simulink model "sla_tf2filter"  (R2015b)
settings: Solver=FixedStepDiscrete  SolverMode=SingleTasking  StartTime=0.0  StopTime=10.0  RelTol=1e-3
undefined symbols (not defined in the file or in its folder): dfilt
libraries: simulink x1, dsparch4 x1
settings Model: Creator=at-mt  LastModifiedBy=amatsumo
settings DataIOCC: SaveFormat=Array  SignalLoggingSaveFormat=ModelDataLogs  SaveOutput=off  SignalLogging=off  SaveTime=off
settings OptimizationCC: BlockReduction=off  ConditionallyExecuteInputs=off  DefaultParameterBehavior=Inlined  ExpressionDepthLimit=2147483647
settings DebuggingCC: AlgebraicLoopMsg=error  UnderspecifiedInitializationDetection=Classic  MergeDetectMultiDrivingBlocksExec=none  SolverPrmCheckMsg=warning  SingleTaskRateTransMsg=error  FcnCallInpInsideContextMsg=UseLocalSettings  StateNameClashWarn=warning
settings HardwareCC: ProdBitPerPointer=32  ProdLargestAtomicFloat=None  ProdIntDivRoundTo=Undefined  ProdEndianess=Unspecified  ProdWordSize=32  ProdHWDeviceType=ASIC/FPGA->ASIC/FPGA  ProdEqTarget=off
settings GRTTargetCC: GeneratePreprocessorConditionals=Disable all  CombineOutputUpdateFcns=off  GRTInterface=on
settings ConfigComp: CovModelRefEnable=Off  CovSFcnEnable=off

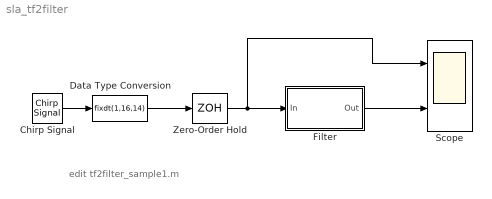
== system sla_tf2filter ==
  note: edit tf2filter_sample1.m
  Chirp Signal : simulink/Sources/Chirp Signal  f1=10  T=10  f2=500
  Data Type Conversion : DataTypeConversion  OutDataTypeStr=fixdt(1,16,14)  RndMeth=Nearest
  Filter : Subsystem  Tag=BlockMethodSubSystem
  Scope : Scope  NumInputPorts=2
  Zero-Order Hold : ZeroOrderHold  SampleTime=1/1000
  wires:
  Chirp Signal/1 -> Data Type Conversion/1
  Zero-Order Hold/1 -> Filter/1(In), Scope/1
  Data Type Conversion/1 -> Zero-Order Hold/1
  Filter/1(Out) -> Scope/2

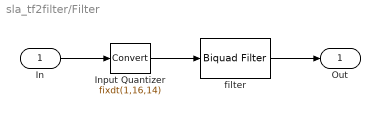
== system sla_tf2filter/Filter ==
  In : Inport
  Input Quantizer : DataTypeConversion  OutDataTypeStr=fixdt(1,16,14)  RndMeth=Round  SaturateOnIntegerOverflow=on
  filter : dsparch4/Biquad Filter  IIRFiltStruct=Direct form I  CoeffSource=Specify via dialog  BiQuadCoeffs=[0.24414136730043 0.246333183206054 0 1 -0.509525449493515 0;0.0620793909084329 0.124857568309846 0.06278319720299 1 -1.05783155795159 0.307551714372856;0.0700184403619336 0.139760096138217 0.0697473544144734 1 -1.18409067538908 0.463616566303708;0.0851377007746378 0.168889277821254 0.0837585371434181 1 -1.43088240648643 0.76866792222576]  a0Flag=Warning  IC=0  ICnum=0  ICden=0  InputProcessing=Inherited (this choice will be removed - see release notes)  firstCoeffMode=Binary point scaling  firstCoeffWordLength=18  firstCoeffFracLength=19  outputMode=Binary point scaling  outputWordLength=16  outputFracLength=14  accumMode=Binary point scaling  accumWordLength=40  accumFracLength=33  denAccumFracLength=30  prodOutputMode=Binary point scaling  prodOutputWordLength=32  prodOutputFracLength=33  denProdOutputFracLength=30  secondMemoryFracLength=15  roundingMode=Convergent  overflowMode=off  ScaleValues=[1;1;1;1;0.999999999999586]  optimizeScaleValues=on  ScaleValueMode=Specify via input port (g)  scaleValueFracLength=17  stageInputMode=Binary point scaling  stageOutputMode=Binary point scaling  stageInputWordLength=16  stageInputFracLength=14  stageOutputWordLength=16  stageOutputFracLength=14  FilterSource=Specify via dialog  FilterObject=dfilt.df2tsos([1 0.3 0.4],[1 0.1 0.2])
  Out : Outport
  wires:
  filter/1 -> Out/1
  Input Quantizer/1 -> filter/1
  In/1 -> Input Quantizer/1
